simulink model "pfb_core_snbxfft"  (R2012b)
settings: Solver=FixedStepDiscrete  SolverMode=SingleTasking  StartTime=0.0  StopTime=5000  FixedStep=1  RelTol=1e-3
undefined symbols (not defined in the file or in its folder): xlipgetpartsetting
undefined symbols (not defined in the file): pfb_coeff_gen_calc
libraries: xbsIndex_r4 x3846, casper_library_misc x2, casper_library_delays x1
(part 4 of 14)

== system pfb_core_snbxfft/pfb/pfb_fir_generic/pfb_fir_coeff_gen/rom ==
  addra : Inport
  dina : Inport  Port=2
  wea : Inport  Port=3
  addrb : Inport  Port=4
  dinb : Inport  Port=5
  web : Inport  Port=6
  A_bussify : Subsystem  AncestorBlock=casper_library_flow_control/bus_create  mask(bus_create){inputNum=18}
      mask prompts: inputNum "Number of inputs:"
      mask init:
      | bus_create_init(gcb,...
      |     'inputNum', inputNum);
  B_bussify : Subsystem  AncestorBlock=casper_library_flow_control/bus_create  mask(bus_create){inputNum=18}
      mask prompts: inputNum "Number of inputs:"
      mask init:
      | bus_create_init(gcb,...
      |     'inputNum', inputNum);
  bram{0..17} (18 alike) : xbsIndex_r4/Dual Port RAM  depth=8192  initVector=getfield(get_param(gcb, 'UserData'), 'initVector')  distributed_mem=Block RAM  init_a=0  init_b=0  rst_a=off  rst_b=off  en_a=off  en_b=off  latency=8  write_mode_A=Read Before Write  write_mode_B=Read Before Write  dbl_ovrd=off  optimize=Speed  block_type=dpram
  ddina : xbsIndex_r4/Delay  rst=off  infoeditControl=Selection of Reset will increase slice count due to use of real FFs and instead of SRLs  en=off  latency=0  dbl_ovrd=off  reg_retiming=on  block_type=delay
  ddinb : xbsIndex_r4/Delay  rst=off  infoeditControl=Selection of Reset will increase slice count due to use of real FFs and instead of SRLs  en=off  latency=0  dbl_ovrd=off  reg_retiming=on  block_type=delay
  debus_addra : Subsystem  AncestorBlock=casper_library_flow_control/bus_expand  mask(bus_expand){mode=divisions of equal size, outputNum=18, outputWidth=[13 13 13 13 13 13 13 13 13 13 13 13 13 13 13 13 13 13], outputBinaryPt=[0 0 0 0 0 0 0 0 0 0 0 0 0 0 0 0 0 0], outputArithmeticType=[0 0 0 0 0 0 0 0 0 0 0 0 0 0 0 0 0 0], show_format=on, outputToWorkspace=off, variablePrefix=, outputToModelAsWell=on}
      mask prompts: outputNum "Number of outputs:"; outputWidth "Output width:"; outputBinaryPt "Output binary point position:"; outputArithmeticType "Output arithmetic type (ufix=0, fix=1, bool=2):"; show_format "Print format string?"; outputToWorkspace "Output to workspace?"; variablePrefix "Variable name prefix:"; outputToModelAsWell "Output to model as well?"
      mask help:
      | Expands a 'bus' made using a bus_create or Xilinx
      | concat block.
      | The input will be divided into the specified number
      | of outputs with the specified arithmetic types.
      | Divisions are made from most significant bit.
      mask init: same as pfb_core_snbxfft/pfb/pfb_fir_generic/bus_expand
      settings: AttributesFormatString=18 outputs: uf13.0,uf13.0,uf13.0,uf13.0,uf13.0,uf13.0,uf13.0,uf13.0,uf13.0,uf13.0,uf13.0,uf13.0,uf13.0,uf13.0,uf13.0,uf13.0,uf13.0,uf13.0,
      mask TypeOptions mode: divisions of equal size | divisions of arbitrary size
      mask Callback mode: bus_expand_callback();
      mask Callback outputWidth: bus_expand_callback();
      mask Callback outputToWorkspace: bus_expand_callback();
  debus_addrb : Subsystem  AncestorBlock=casper_library_flow_control/bus_expand  mask(bus_expand){mode=divisions of equal size, outputNum=18, outputWidth=[13 13 13 13 13 13 13 13 13 13 13 13 13 13 13 13 13 13], outputBinaryPt=[0 0 0 0 0 0 0 0 0 0 0 0 0 0 0 0 0 0], outputArithmeticType=[0 0 0 0 0 0 0 0 0 0 0 0 0 0 0 0 0 0], show_format=on, outputToWorkspace=off, variablePrefix=, outputToModelAsWell=on}
      mask prompts: outputNum "Number of outputs:"; outputWidth "Output width:"; outputBinaryPt "Output binary point position:"; outputArithmeticType "Output arithmetic type (ufix=0, fix=1, bool=2):"; show_format "Print format string?"; outputToWorkspace "Output to workspace?"; variablePrefix "Variable name prefix:"; outputToModelAsWell "Output to model as well?"
      mask help:
      | Expands a 'bus' made using a bus_create or Xilinx
      | concat block.
      | The input will be divided into the specified number
      | of outputs with the specified arithmetic types.
      | Divisions are made from most significant bit.
      mask init: same as pfb_core_snbxfft/pfb/pfb_fir_generic/bus_expand
      settings: AttributesFormatString=18 outputs: uf13.0,uf13.0,uf13.0,uf13.0,uf13.0,uf13.0,uf13.0,uf13.0,uf13.0,uf13.0,uf13.0,uf13.0,uf13.0,uf13.0,uf13.0,uf13.0,uf13.0,uf13.0,
      mask TypeOptions mode: divisions of equal size | divisions of arbitrary size
      mask Callback mode: bus_expand_callback();
      mask Callback outputWidth: bus_expand_callback();
      mask Callback outputToWorkspace: bus_expand_callback();
  debus_dina : Subsystem  AncestorBlock=casper_library_flow_control/bus_expand  mask(bus_expand){mode=divisions of arbitrary size, outputNum=1, outputWidth=[4 4 4 4 4 4 4 4 4 4 4 4 4 4 4 4 4 4], outputBinaryPt=[0 0 0 0 0 0 0 0 0 0 0 0 0 0 0 0 0 0], outputArithmeticType=[0 0 0 0 0 0 0 0 0 0 0 0 0 0 0 0 0 0], show_format=on, outputToWorkspace=off, variablePrefix=, outputToModelAsWell=on}
      mask prompts: outputNum "Number of outputs:"; outputWidth "Output width [msb ... lsb]:"; outputBinaryPt "Output binary point position [msb ... lsb]:"; outputArithmeticType "Output arithmetic type (ufix=0, fix=1, bool=2) [msb ... lsb]:"; show_format "Print format string?"; outputToWorkspace "Output to workspace?"; variablePrefix "Variable name prefix:"; outputToModelAsWell "Output to model as well?"
      mask help:
      | Expands a 'bus' made using a bus_create or Xilinx
      | concat block.
      | The input will be divided into the specified number
      | of outputs with the specified arithmetic types.
      | Divisions are made from most significant bit.
      mask init: same as pfb_core_snbxfft/pfb/pfb_fir_generic/bus_expand
      settings: AttributesFormatString=18 outputs: uf4.0,uf4.0,uf4.0,uf4.0,uf4.0,uf4.0,uf4.0,uf4.0,uf4.0,uf4.0,uf4.0,uf4.0,uf4.0,uf4.0,uf4.0,uf4.0,uf4.0,uf4.0,
      mask TypeOptions mode: divisions of equal size | divisions of arbitrary size
      mask Callback mode: bus_expand_callback();
      mask Callback outputWidth: bus_expand_callback();
      mask Callback outputToWorkspace: bus_expand_callback();
  debus_dinb : Subsystem  AncestorBlock=casper_library_flow_control/bus_expand  mask(bus_expand){mode=divisions of arbitrary size, outputNum=1, outputWidth=[4 4 4 4 4 4 4 4 4 4 4 4 4 4 4 4 4 4], outputBinaryPt=[0 0 0 0 0 0 0 0 0 0 0 0 0 0 0 0 0 0], outputArithmeticType=[0 0 0 0 0 0 0 0 0 0 0 0 0 0 0 0 0 0], show_format=on, outputToWorkspace=off, variablePrefix=, outputToModelAsWell=on}
      mask prompts: outputNum "Number of outputs:"; outputWidth "Output width [msb ... lsb]:"; outputBinaryPt "Output binary point position [msb ... lsb]:"; outputArithmeticType "Output arithmetic type (ufix=0, fix=1, bool=2) [msb ... lsb]:"; show_format "Print format string?"; outputToWorkspace "Output to workspace?"; variablePrefix "Variable name prefix:"; outputToModelAsWell "Output to model as well?"
      mask help:
      | Expands a 'bus' made using a bus_create or Xilinx
      | concat block.
      | The input will be divided into the specified number
      | of outputs with the specified arithmetic types.
      | Divisions are made from most significant bit.
      mask init: same as pfb_core_snbxfft/pfb/pfb_fir_generic/bus_expand
      settings: AttributesFormatString=18 outputs: uf4.0,uf4.0,uf4.0,uf4.0,uf4.0,uf4.0,uf4.0,uf4.0,uf4.0,uf4.0,uf4.0,uf4.0,uf4.0,uf4.0,uf4.0,uf4.0,uf4.0,uf4.0,
      mask TypeOptions mode: divisions of equal size | divisions of arbitrary size
      mask Callback mode: bus_expand_callback();
      mask Callback outputWidth: bus_expand_callback();
      mask Callback outputToWorkspace: bus_expand_callback();
  debus_wea : Subsystem  AncestorBlock=casper_library_flow_control/bus_expand  mask(bus_expand){mode=divisions of equal size, outputNum=18, outputWidth=[1 1 1 1 1 1 1 1 1 1 1 1 1 1 1 1 1 1], outputBinaryPt=[0 0 0 0 0 0 0 0 0 0 0 0 0 0 0 0 0 0], outputArithmeticType=[2 2 2 2 2 2 2 2 2 2 2 2 2 2 2 2 2 2], show_format=on, outputToWorkspace=off, variablePrefix=, outputToModelAsWell=on}
      mask prompts: outputNum "Number of outputs:"; outputWidth "Output width:"; outputBinaryPt "Output binary point position:"; outputArithmeticType "Output arithmetic type (ufix=0, fix=1, bool=2):"; show_format "Print format string?"; outputToWorkspace "Output to workspace?"; variablePrefix "Variable name prefix:"; outputToModelAsWell "Output to model as well?"
      mask help:
      | Expands a 'bus' made using a bus_create or Xilinx
      | concat block.
      | The input will be divided into the specified number
      | of outputs with the specified arithmetic types.
      | Divisions are made from most significant bit.
      mask init: same as pfb_core_snbxfft/pfb/pfb_fir_generic/bus_expand
      settings: AttributesFormatString=18 outputs: b,b,b,b,b,b,b,b,b,b,b,b,b,b,b,b,b,b,
      mask TypeOptions mode: divisions of equal size | divisions of arbitrary size
      mask Callback mode: bus_expand_callback();
      mask Callback outputWidth: bus_expand_callback();
      mask Callback outputToWorkspace: bus_expand_callback();
  debus_web : Subsystem  AncestorBlock=casper_library_flow_control/bus_expand  mask(bus_expand){mode=divisions of equal size, outputNum=18, outputWidth=[1 1 1 1 1 1 1 1 1 1 1 1 1 1 1 1 1 1], outputBinaryPt=[0 0 0 0 0 0 0 0 0 0 0 0 0 0 0 0 0 0], outputArithmeticType=[2 2 2 2 2 2 2 2 2 2 2 2 2 2 2 2 2 2], show_format=on, outputToWorkspace=off, variablePrefix=, outputToModelAsWell=on}
      mask prompts: outputNum "Number of outputs:"; outputWidth "Output width:"; outputBinaryPt "Output binary point position:"; outputArithmeticType "Output arithmetic type (ufix=0, fix=1, bool=2):"; show_format "Print format string?"; outputToWorkspace "Output to workspace?"; variablePrefix "Variable name prefix:"; outputToModelAsWell "Output to model as well?"
      mask help:
      | Expands a 'bus' made using a bus_create or Xilinx
      | concat block.
      | The input will be divided into the specified number
      | of outputs with the specified arithmetic types.
      | Divisions are made from most significant bit.
      mask init: same as pfb_core_snbxfft/pfb/pfb_fir_generic/bus_expand
      settings: AttributesFormatString=18 outputs: b,b,b,b,b,b,b,b,b,b,b,b,b,b,b,b,b,b,
      mask TypeOptions mode: divisions of equal size | divisions of arbitrary size
      mask Callback mode: bus_expand_callback();
      mask Callback outputWidth: bus_expand_callback();
      mask Callback outputToWorkspace: bus_expand_callback();
  rep_addra : Subsystem  AncestorBlock=casper_library_bus/bus_replicate  mask(bus_replicate){replication=18, latency=9, misc=off, implementation=core}
      mask prompts: replication "replication factor"; misc "misc support"; implementation "delay implementation"
      mask help: Output bus formed by replicating input bus a number of times
      mask init:
      | bus_replicate_init(gcb, ...
      |     'replication', replication, ...
      |     'latency', latency, ...
      |     'implementation', implementation, ...
      |     'misc', misc);
      mask TypeOptions implementation: core | behavioral
  rep_addrb : Subsystem  AncestorBlock=casper_library_bus/bus_replicate  mask(bus_replicate){replication=18, latency=9, misc=off, implementation=core}
      mask prompts: replication "replication factor"; misc "misc support"; implementation "delay implementation"
      mask help: Output bus formed by replicating input bus a number of times
      mask init:
      | bus_replicate_init(gcb, ...
      |     'replication', replication, ...
      |     'latency', latency, ...
      |     'implementation', implementation, ...
      |     'misc', misc);
      mask TypeOptions implementation: core | behavioral
  rep_wea : Subsystem  AncestorBlock=casper_library_bus/bus_replicate  mask(bus_replicate){replication=18, latency=0, misc=off, implementation=behavioral}
      mask prompts: replication "replication factor"; misc "misc support"; implementation "delay implementation"
      mask help: Output bus formed by replicating input bus a number of times
      mask init:
      | bus_replicate_init(gcb, ...
      |     'replication', replication, ...
      |     'latency', latency, ...
      |     'implementation', implementation, ...
      |     'misc', misc);
      mask TypeOptions implementation: core | behavioral
  rep_web : Subsystem  AncestorBlock=casper_library_bus/bus_replicate  mask(bus_replicate){replication=18, latency=0, misc=off, implementation=behavioral}
      mask prompts: replication "replication factor"; misc "misc support"; implementation "delay implementation"
      mask help: Output bus formed by replicating input bus a number of times
      mask init:
      | bus_replicate_init(gcb, ...
      |     'replication', replication, ...
      |     'latency', latency, ...
      |     'implementation', implementation, ...
      |     'misc', misc);
      mask TypeOptions implementation: core | behavioral
  A : Outport
  B : Outport  Port=2
  wires:
  addra/1 -> rep_addra/1(in)
  dina/1 -> ddina/1
  wea/1 -> rep_wea/1(in)
  addrb/1 -> rep_addrb/1(in)
  dinb/1 -> ddinb/1
  web/1 -> rep_web/1(in)
  rep_addra/1(out) -> debus_addra/1(bus_in)
  ddina/1 -> debus_dina/1(bus_in)
  rep_wea/1(out) -> debus_wea/1(bus_in)
  rep_addrb/1(out) -> debus_addrb/1(bus_in)
  ddinb/1 -> debus_dinb/1(bus_in)
  rep_web/1(out) -> debus_web/1(bus_in)
  debus_addra/1(msb_out18) -> bram0/1
  debus_dina/1(msb_out18) -> bram0/2
  debus_wea/1(msb_out18) -> bram0/3
  debus_addrb/1(msb_out18) -> bram0/4
  debus_dinb/1(msb_out18) -> bram0/5
  debus_web/1(msb_out18) -> bram0/6
  debus_addra/2(out17) -> bram1/1
  debus_dina/2(out17) -> bram1/2
  debus_wea/2(out17) -> bram1/3
  debus_addrb/2(out17) -> bram1/4
  debus_dinb/2(out17) -> bram1/5
  debus_web/2(out17) -> bram1/6
  debus_addra/3(out16) -> bram2/1
  debus_dina/3(out16) -> bram2/2
  debus_wea/3(out16) -> bram2/3
  debus_addrb/3(out16) -> bram2/4
  debus_dinb/3(out16) -> bram2/5
  debus_web/3(out16) -> bram2/6
  debus_addra/4(out15) -> bram3/1
  debus_dina/4(out15) -> bram3/2
  debus_wea/4(out15) -> bram3/3
  debus_addrb/4(out15) -> bram3/4
  debus_dinb/4(out15) -> bram3/5
  debus_web/4(out15) -> bram3/6
  debus_addra/5(out14) -> bram4/1
  debus_dina/5(out14) -> bram4/2
  debus_wea/5(out14) -> bram4/3
  debus_addrb/5(out14) -> bram4/4
  debus_dinb/5(out14) -> bram4/5
  debus_web/5(out14) -> bram4/6
  debus_addra/6(out13) -> bram5/1
  debus_dina/6(out13) -> bram5/2
  debus_wea/6(out13) -> bram5/3
  debus_addrb/6(out13) -> bram5/4
  debus_dinb/6(out13) -> bram5/5
  debus_web/6(out13) -> bram5/6
  debus_addra/7(out12) -> bram6/1
  debus_dina/7(out12) -> bram6/2
  debus_wea/7(out12) -> bram6/3
  debus_addrb/7(out12) -> bram6/4
  debus_dinb/7(out12) -> bram6/5
  debus_web/7(out12) -> bram6/6
  debus_addra/8(out11) -> bram7/1
  debus_dina/8(out11) -> bram7/2
  debus_wea/8(out11) -> bram7/3
  debus_addrb/8(out11) -> bram7/4
  debus_dinb/8(out11) -> bram7/5
  debus_web/8(out11) -> bram7/6
  debus_addra/9(out10) -> bram8/1
  debus_dina/9(out10) -> bram8/2
  debus_wea/9(out10) -> bram8/3
  debus_addrb/9(out10) -> bram8/4
  debus_dinb/9(out10) -> bram8/5
  debus_web/9(out10) -> bram8/6
  debus_addra/10(out9) -> bram9/1
  debus_dina/10(out9) -> bram9/2
  debus_wea/10(out9) -> bram9/3
  debus_addrb/10(out9) -> bram9/4
  debus_dinb/10(out9) -> bram9/5
  debus_web/10(out9) -> bram9/6
  debus_addra/11(out8) -> bram10/1
  debus_dina/11(out8) -> bram10/2
  debus_wea/11(out8) -> bram10/3
  debus_addrb/11(out8) -> bram10/4
  debus_dinb/11(out8) -> bram10/5
  debus_web/11(out8) -> bram10/6
  debus_addra/12(out7) -> bram11/1
  debus_dina/12(out7) -> bram11/2
  debus_wea/12(out7) -> bram11/3
  debus_addrb/12(out7) -> bram11/4
  debus_dinb/12(out7) -> bram11/5
  debus_web/12(out7) -> bram11/6
  debus_addra/13(out6) -> bram12/1
  debus_dina/13(out6) -> bram12/2
  debus_wea/13(out6) -> bram12/3
  debus_addrb/13(out6) -> bram12/4
  debus_dinb/13(out6) -> bram12/5
  debus_web/13(out6) -> bram12/6
  debus_addra/14(out5) -> bram13/1
  debus_dina/14(out5) -> bram13/2
  debus_wea/14(out5) -> bram13/3
  debus_addrb/14(out5) -> bram13/4
  debus_dinb/14(out5) -> bram13/5
  debus_web/14(out5) -> bram13/6
  debus_addra/15(out4) -> bram14/1
  debus_dina/15(out4) -> bram14/2
  debus_wea/15(out4) -> bram14/3
  debus_addrb/15(out4) -> bram14/4
  debus_dinb/15(out4) -> bram14/5
  debus_web/15(out4) -> bram14/6
  debus_addra/16(out3) -> bram15/1
  debus_dina/16(out3) -> bram15/2
  debus_wea/16(out3) -> bram15/3
  debus_addrb/16(out3) -> bram15/4
  debus_dinb/16(out3) -> bram15/5
  debus_web/16(out3) -> bram15/6
  debus_addra/17(out2) -> bram16/1
  debus_dina/17(out2) -> bram16/2
  debus_wea/17(out2) -> bram16/3
  debus_addrb/17(out2) -> bram16/4
  debus_dinb/17(out2) -> bram16/5
  debus_web/17(out2) -> bram16/6
  debus_addra/18(lsb_out1) -> bram17/1
  debus_dina/18(lsb_out1) -> bram17/2
  debus_wea/18(lsb_out1) -> bram17/3
  debus_addrb/18(lsb_out1) -> bram17/4
  debus_dinb/18(lsb_out1) -> bram17/5
  debus_web/18(lsb_out1) -> bram17/6
  bram0/1 -> A_bussify/1(in1)
  bram0/2 -> B_bussify/1(in1)
  bram1/1 -> A_bussify/2(in2)
  bram1/2 -> B_bussify/2(in2)
  bram2/1 -> A_bussify/3(in3)
  bram2/2 -> B_bussify/3(in3)
  bram3/1 -> A_bussify/4(in4)
  bram3/2 -> B_bussify/4(in4)
  bram4/1 -> A_bussify/5(in5)
  bram4/2 -> B_bussify/5(in5)
  bram5/1 -> A_bussify/6(in6)
  bram5/2 -> B_bussify/6(in6)
  bram6/1 -> A_bussify/7(in7)
  bram6/2 -> B_bussify/7(in7)
  bram7/1 -> A_bussify/8(in8)
  bram7/2 -> B_bussify/8(in8)
  bram8/1 -> A_bussify/9(in9)
  bram8/2 -> B_bussify/9(in9)
  bram9/1 -> A_bussify/10(in10)
  bram9/2 -> B_bussify/10(in10)
  bram10/1 -> A_bussify/11(in11)
  bram10/2 -> B_bussify/11(in11)
  bram11/1 -> A_bussify/12(in12)
  bram11/2 -> B_bussify/12(in12)
  bram12/1 -> A_bussify/13(in13)
  bram12/2 -> B_bussify/13(in13)
  bram13/1 -> A_bussify/14(in14)
  bram13/2 -> B_bussify/14(in14)
  bram14/1 -> A_bussify/15(in15)
  bram14/2 -> B_bussify/15(in15)
  bram15/1 -> A_bussify/16(in16)
  bram15/2 -> B_bussify/16(in16)
  bram16/1 -> A_bussify/17(in17)
  bram16/2 -> B_bussify/17(in17)
  bram17/1 -> A_bussify/18(in18)
  bram17/2 -> B_bussify/18(in18)
  A_bussify/1(bus_out) -> A/1
  B_bussify/1(bus_out) -> B/1

== system pfb_core_snbxfft/pfb/pfb_fir_generic/pfb_fir_taps/bus_madd ==
  a : Inport
  b : Inport  Port=2
  c : Inport  Port=3
  en : Inport  Port=4
  a*b+c_bussify : Subsystem  AncestorBlock=casper_library_flow_control/bus_create  mask(bus_create){inputNum=32}
      mask prompts: inputNum "Number of inputs:"
      mask init:
      | bus_create_init(gcb,...
      |     'inputNum', inputNum);
  a_debus : Subsystem  AncestorBlock=casper_library_flow_control/bus_expand  mask(bus_expand){mode=divisions of arbitrary size, outputNum=1, outputWidth=[18 18 18 18 18 18 18 18 18 18 18 18 18 18 18 18 18 18 18 18 18 18 18 18 18 18 18 18 18 18 18 18], outputBinaryPt=[17 17 17 17 17 17 17 17 17 17 17 17 17 17 17 17 17 17 17 17 17 17 17 17 17 17 17 17 17 17 17 17], outputArithmeticType=[1 1 1 1 1 1 1 1 1 1 1 1 1 1 1 1 1 1 1 1 1 1 1 1 1 1 1 1 1 1 1 1], show_format=on, outputToWorkspace=off, variablePrefix=, outputToModelAsWell=on}
      mask prompts: outputNum "Number of outputs:"; outputWidth "Output width [msb ... lsb]:"; outputBinaryPt "Output binary point position [msb ... lsb]:"; outputArithmeticType "Output arithmetic type (ufix=0, fix=1, bool=2) [msb ... lsb]:"; show_format "Print format string?"; outputToWorkspace "Output to workspace?"; variablePrefix "Variable name prefix:"; outputToModelAsWell "Output to model as well?"
      mask help:
      | Expands a 'bus' made using a bus_create or Xilinx
      | concat block.
      | The input will be divided into the specified number
      | of outputs with the specified arithmetic types.
      | Divisions are made from most significant bit.
      mask init: same as pfb_core_snbxfft/pfb/pfb_fir_generic/bus_expand
      settings: AttributesFormatString=32 outputs: f18.17,f18.17,f18.17,f18.17,f18.17,f18.17,f18.17,f18.17,f18.17,f18.17,f18.17,f18.17,f18.17,f18.17,f18.17,f18.17,f18.17,f18.17,f18.17,f18.17,f18.17,f18.17,f18.17,f18.17,f18.17,f18.17,f18.17,f18.17,f18.17,f18.17,f18.17,f18.17,
      mask TypeOptions mode: divisions of equal size | divisions of arbitrary size
      mask Callback mode: bus_expand_callback();
      mask Callback outputWidth: bus_expand_callback();
      mask Callback outputToWorkspace: bus_expand_callback();
  addsub{1..4} (4 alike) : xbsIndex_r4/AddSub  mode=Addition  use_carryin=off  use_carryout=off  en=on  latency=2  precision=User Defined  arith_type="Signed  (2's comp)"  n_bits=36  bin_pt=34  quantization=Truncate  overflow=Wrap  dbl_ovrd=off  use_behavioral_HDL=on  hw_selection=Fabric  pipelined=on  block_type=addsub
  addsub{9..12} (4 alike) : xbsIndex_r4/AddSub  mode=Addition  use_carryin=off  use_carryout=off  en=on  latency=2  precision=User Defined  arith_type="Signed  (2's comp)"  n_bits=38  bin_pt=34  quantization=Truncate  overflow=Wrap  dbl_ovrd=off  use_behavioral_HDL=on  hw_selection=Fabric  pipelined=on  block_type=addsub
  addsub{13..16} (4 alike) : xbsIndex_r4/AddSub  mode=Addition  use_carryin=off  use_carryout=off  en=on  latency=2  precision=User Defined  arith_type="Signed  (2's comp)"  n_bits=39  bin_pt=34  quantization=Truncate  overflow=Wrap  dbl_ovrd=off  use_behavioral_HDL=on  hw_selection=Fabric  pipelined=on  block_type=addsub
  addsub{17..20} (4 alike) : xbsIndex_r4/AddSub  mode=Addition  use_carryin=off  use_carryout=off  en=on  latency=2  precision=User Defined  arith_type="Signed  (2's comp)"  n_bits=40  bin_pt=34  quantization=Truncate  overflow=Wrap  dbl_ovrd=off  use_behavioral_HDL=on  hw_selection=Fabric  pipelined=on  block_type=addsub
  addsub{21..24} (4 alike) : xbsIndex_r4/AddSub  mode=Addition  use_carryin=off  use_carryout=off  en=on  latency=2  precision=User Defined  arith_type="Signed  (2's comp)"  n_bits=41  bin_pt=34  quantization=Truncate  overflow=Wrap  dbl_ovrd=off  use_behavioral_HDL=on  hw_selection=Fabric  pipelined=on  block_type=addsub
  addsub{25..28} (4 alike) : xbsIndex_r4/AddSub  mode=Addition  use_carryin=off  use_carryout=off  en=on  latency=2  precision=User Defined  arith_type="Signed  (2's comp)"  n_bits=42  bin_pt=34  quantization=Truncate  overflow=Wrap  dbl_ovrd=off  use_behavioral_HDL=on  hw_selection=Fabric  pipelined=on  block_type=addsub
  addsub{29..32} (4 alike) : xbsIndex_r4/AddSub  mode=Addition  use_carryin=off  use_carryout=off  en=on  latency=2  precision=User Defined  arith_type="Signed  (2's comp)"  n_bits=43  bin_pt=34  quantization=Truncate  overflow=Wrap  dbl_ovrd=off  use_behavioral_HDL=on  hw_selection=Fabric  pipelined=on  block_type=addsub
  addsub{5..8} (4 alike) : xbsIndex_r4/AddSub  mode=Addition  use_carryin=off  use_carryout=off  en=on  latency=2  precision=User Defined  arith_type="Signed  (2's comp)"  n_bits=37  bin_pt=34  quantization=Truncate  overflow=Wrap  dbl_ovrd=off  use_behavioral_HDL=on  hw_selection=Fabric  pipelined=on  block_type=addsub
  b_debus : Subsystem  AncestorBlock=casper_library_flow_control/bus_expand  mask(bus_expand){mode=divisions of arbitrary size, outputNum=1, outputWidth=[18 18 18 18 18 18 18 18 18 18 18 18 18 18 18 18 18 18 18 18 18 18 18 18 18 18 18 18 18 18 18 18], outputBinaryPt=[17 17 17 17 17 17 17 17 17 17 17 17 17 17 17 17 17 17 17 17 17 17 17 17 17 17 17 17 17 17 17 17], outputArithmeticType=[1 1 1 1 1 1 1 1 1 1 1 1 1 1 1 1 1 1 1 1 1 1 1 1 1 1 1 1 1 1 1 1], show_format=on, outputToWorkspace=off, variablePrefix=, outputToModelAsWell=on}
      mask prompts: outputNum "Number of outputs:"; outputWidth "Output width [msb ... lsb]:"; outputBinaryPt "Output binary point position [msb ... lsb]:"; outputArithmeticType "Output arithmetic type (ufix=0, fix=1, bool=2) [msb ... lsb]:"; show_format "Print format string?"; outputToWorkspace "Output to workspace?"; variablePrefix "Variable name prefix:"; outputToModelAsWell "Output to model as well?"
      mask help:
      | Expands a 'bus' made using a bus_create or Xilinx
      | concat block.
      | The input will be divided into the specified number
      | of outputs with the specified arithmetic types.
      | Divisions are made from most significant bit.
      mask init: same as pfb_core_snbxfft/pfb/pfb_fir_generic/bus_expand
      settings: AttributesFormatString=32 outputs: f18.17,f18.17,f18.17,f18.17,f18.17,f18.17,f18.17,f18.17,f18.17,f18.17,f18.17,f18.17,f18.17,f18.17,f18.17,f18.17,f18.17,f18.17,f18.17,f18.17,f18.17,f18.17,f18.17,f18.17,f18.17,f18.17,f18.17,f18.17,f18.17,f18.17,f18.17,f18.17,
      mask TypeOptions mode: divisions of equal size | divisions of arbitrary size
      mask Callback mode: bus_expand_callback();
      mask Callback outputWidth: bus_expand_callback();
      mask Callback outputToWorkspace: bus_expand_callback();
  c_debus : Subsystem  AncestorBlock=casper_library_flow_control/bus_expand  mask(bus_expand){mode=divisions of arbitrary size, outputNum=1, outputWidth=[36 36 36 36 36 36 36 36 37 37 37 37 38 38 38 38 39 39 39 39 40 40 40 40 41 41 41 41 42 42 42 42], outputBinaryPt=[34 34 34 34 34 34 34 34 34 34 34 34 34 34 34 34 34 34 34 34 34 34 34 34 34 34 34 34 34 34 34 34], outputArithmeticType=[1 1 1 1 1 1 1 1 1 1 1 1 1 1 1 1 1 1 1 1 1 1 1 1 1 1 1 1 1 1 1 1], show_format=on, outputToWorkspace=off, variablePrefix=, outputToModelAsWell=on}
      mask prompts: outputNum "Number of outputs:"; outputWidth "Output width [msb ... lsb]:"; outputBinaryPt "Output binary point position [msb ... lsb]:"; outputArithmeticType "Output arithmetic type (ufix=0, fix=1, bool=2) [msb ... lsb]:"; show_format "Print format string?"; outputToWorkspace "Output to workspace?"; variablePrefix "Variable name prefix:"; outputToModelAsWell "Output to model as well?"
      mask help:
      | Expands a 'bus' made using a bus_create or Xilinx
      | concat block.
      | The input will be divided into the specified number
      | of outputs with the specified arithmetic types.
      | Divisions are made from most significant bit.
      mask init: same as pfb_core_snbxfft/pfb/pfb_fir_generic/bus_expand
      settings: AttributesFormatString=32 outputs: f36.34,f36.34,f36.34,f36.34,f36.34,f36.34,f36.34,f36.34,f37.34,f37.34,f37.34,f37.34,f38.34,f38.34,f38.34,f38.34,f39.34,f39.34,f39.34,f39.34,f40.34,f40.34,f40.34,f40.34,f41.34,f41.34,f41.34,f41.34,f42.34,f42.34,f42.34,f42.34,
      mask TypeOptions mode: divisions of equal size | divisions of arbitrary size
      mask Callback mode: bus_expand_callback();
      mask Callback outputWidth: bus_expand_callback();
      mask Callback outputToWorkspace: bus_expand_callback();
  den0 : xbsIndex_r4/Delay  rst=off  infoeditControl=Selection of Reset will increase slice count due to use of real FFs and instead of SRLs  en=off  latency=3  dbl_ovrd=off  reg_retiming=on  block_type=delay
  den1 : xbsIndex_r4/Delay  rst=off  infoeditControl=Selection of Reset will increase slice count due to use of real FFs and instead of SRLs  en=off  latency=1  dbl_ovrd=off  reg_retiming=on  block_type=delay
  den2 : xbsIndex_r4/Delay  rst=off  infoeditControl=Selection of Reset will increase slice count due to use of real FFs and instead of SRLs  en=off  latency=2  dbl_ovrd=off  reg_retiming=on  block_type=delay
  en_debus1 : Subsystem  AncestorBlock=casper_library_flow_control/bus_expand  mask(bus_expand){mode=divisions of equal size, outputNum=32, outputWidth=1, outputBinaryPt=0, outputArithmeticType=2, show_format=on, outputToWorkspace=off, variablePrefix=, outputToModelAsWell=on}
      mask prompts: outputNum "Number of outputs:"; outputWidth "Output width:"; outputBinaryPt "Output binary point position:"; outputArithmeticType "Output arithmetic type (ufix=0, fix=1, bool=2):"; show_format "Print format string?"; outputToWorkspace "Output to workspace?"; variablePrefix "Variable name prefix:"; outputToModelAsWell "Output to model as well?"
      mask help:
      | Expands a 'bus' made using a bus_create or Xilinx
      | concat block.
      | The input will be divided into the specified number
      | of outputs with the specified arithmetic types.
      | Divisions are made from most significant bit.
      mask init: same as pfb_core_snbxfft/pfb/pfb_fir_generic/bus_expand
      settings: AttributesFormatString=32 outputs: b,b,b,b,b,b,b,b,b,b,b,b,b,b,b,b,b,b,b,b,b,b,b,b,b,b,b,b,b,b,b,b,
      mask TypeOptions mode: divisions of equal size | divisions of arbitrary size
      mask Callback mode: bus_expand_callback();
      mask Callback outputWidth: bus_expand_callback();
      mask Callback outputToWorkspace: bus_expand_callback();
  mult{1..32} (32 alike) : xbsIndex_r4/Mult  precision=Full  arith_type="Signed  (2's comp)"  n_bits=16  bin_pt=14  quantization=Truncate  overflow=Wrap  en=off  latency=3  dbl_ovrd=off  use_behavioral_HDL=on  opt=Speed  use_embedded=off  optimum_pipeline=off  pipeline=on  use_rpm=on  placement_style=Triangular  block_type=mult
  repa : Subsystem  AncestorBlock=casper_library_bus/bus_replicate  mask(bus_replicate){replication=1, latency=1, misc=off, implementation=core}
      mask prompts: replication "replication factor"; misc "misc support"; implementation "delay implementation"
      mask help: Output bus formed by replicating input bus a number of times
      mask init:
      | bus_replicate_init(gcb, ...
      |     'replication', replication, ...
      |     'latency', latency, ...
      |     'implementation', implementation, ...
      |     'misc', misc);
      mask TypeOptions implementation: core | behavioral
  repb : Subsystem  AncestorBlock=casper_library_bus/bus_replicate  mask(bus_replicate){replication=1, latency=1, misc=off, implementation=core}
      mask prompts: replication "replication factor"; misc "misc support"; implementation "delay implementation"
      mask help: Output bus formed by replicating input bus a number of times
      mask init:
      | bus_replicate_init(gcb, ...
      |     'replication', replication, ...
      |     'latency', latency, ...
      |     'implementation', implementation, ...
      |     'misc', misc);
      mask TypeOptions implementation: core | behavioral
  repen1 : Subsystem  AncestorBlock=casper_library_bus/bus_replicate  mask(bus_replicate){replication=32, latency=4, misc=off, implementation=core}
      mask prompts: replication "replication factor"; misc "misc support"; implementation "delay implementation"
      mask help: Output bus formed by replicating input bus a number of times
      mask init:
      | bus_replicate_init(gcb, ...
      |     'replication', replication, ...
      |     'latency', latency, ...
      |     'implementation', implementation, ...
      |     'misc', misc);
      mask TypeOptions implementation: core | behavioral
  a*b+c : Outport
  dvalid : Outport  Port=2
  wires:
  den2/1 -> dvalid/1
  a*b+c_bussify/1(bus_out) -> a*b+c/1
  addsub32/1 -> a*b+c_bussify/32(in32)
  addsub31/1 -> a*b+c_bussify/31(in31)
  addsub30/1 -> a*b+c_bussify/30(in30)
  addsub29/1 -> a*b+c_bussify/29(in29)
  addsub28/1 -> a*b+c_bussify/28(in28)
  addsub27/1 -> a*b+c_bussify/27(in27)
  addsub26/1 -> a*b+c_bussify/26(in26)
  addsub25/1 -> a*b+c_bussify/25(in25)
  addsub24/1 -> a*b+c_bussify/24(in24)
  addsub23/1 -> a*b+c_bussify/23(in23)
  addsub22/1 -> a*b+c_bussify/22(in22)
  addsub21/1 -> a*b+c_bussify/21(in21)
  addsub20/1 -> a*b+c_bussify/20(in20)
  addsub19/1 -> a*b+c_bussify/19(in19)
  addsub18/1 -> a*b+c_bussify/18(in18)
  addsub17/1 -> a*b+c_bussify/17(in17)
  addsub16/1 -> a*b+c_bussify/16(in16)
  addsub15/1 -> a*b+c_bussify/15(in15)
  addsub14/1 -> a*b+c_bussify/14(in14)
  addsub13/1 -> a*b+c_bussify/13(in13)
  addsub12/1 -> a*b+c_bussify/12(in12)
  addsub11/1 -> a*b+c_bussify/11(in11)
  addsub10/1 -> a*b+c_bussify/10(in10)
  addsub9/1 -> a*b+c_bussify/9(in9)
  addsub8/1 -> a*b+c_bussify/8(in8)
  addsub7/1 -> a*b+c_bussify/7(in7)
  addsub6/1 -> a*b+c_bussify/6(in6)
  addsub5/1 -> a*b+c_bussify/5(in5)
  addsub4/1 -> a*b+c_bussify/4(in4)
  addsub3/1 -> a*b+c_bussify/3(in3)
  addsub2/1 -> a*b+c_bussify/2(in2)
  addsub1/1 -> a*b+c_bussify/1(in1)
  den1/1 -> den2/1
  en_debus1/32(lsb_out1) -> addsub32/3
  c_debus/32(lsb_out1) -> addsub32/2
  mult32/1 -> addsub32/1
  en_debus1/31(out2) -> addsub31/3
  c_debus/31(out2) -> addsub31/2
  mult31/1 -> addsub31/1
  en_debus1/30(out3) -> addsub30/3
  c_debus/30(out3) -> addsub30/2
  mult30/1 -> addsub30/1
  en_debus1/29(out4) -> addsub29/3
  c_debus/29(out4) -> addsub29/2
  mult29/1 -> addsub29/1
  en_debus1/28(out5) -> addsub28/3
  c_debus/28(out5) -> addsub28/2
  mult28/1 -> addsub28/1
  en_debus1/27(out6) -> addsub27/3
  c_debus/27(out6) -> addsub27/2
  mult27/1 -> addsub27/1
  en_debus1/26(out7) -> addsub26/3
  c_debus/26(out7) -> addsub26/2
  mult26/1 -> addsub26/1
  en_debus1/25(out8) -> addsub25/3
  c_debus/25(out8) -> addsub25/2
  mult25/1 -> addsub25/1
  en_debus1/24(out9) -> addsub24/3
  c_debus/24(out9) -> addsub24/2
  mult24/1 -> addsub24/1
  en_debus1/23(out10) -> addsub23/3
  c_debus/23(out10) -> addsub23/2
  mult23/1 -> addsub23/1
  en_debus1/22(out11) -> addsub22/3
  c_debus/22(out11) -> addsub22/2
  mult22/1 -> addsub22/1
  en_debus1/21(out12) -> addsub21/3
  c_debus/21(out12) -> addsub21/2
  mult21/1 -> addsub21/1
  en_debus1/20(out13) -> addsub20/3
  c_debus/20(out13) -> addsub20/2
  mult20/1 -> addsub20/1
  en_debus1/19(out14) -> addsub19/3
  c_debus/19(out14) -> addsub19/2
  mult19/1 -> addsub19/1
  en_debus1/18(out15) -> addsub18/3
  c_debus/18(out15) -> addsub18/2
  mult18/1 -> addsub18/1
  en_debus1/17(out16) -> addsub17/3
  c_debus/17(out16) -> addsub17/2
  mult17/1 -> addsub17/1
  en_debus1/16(out17) -> addsub16/3
  c_debus/16(out17) -> addsub16/2
  mult16/1 -> addsub16/1
  en_debus1/15(out18) -> addsub15/3
  c_debus/15(out18) -> addsub15/2
  mult15/1 -> addsub15/1
  en_debus1/14(out19) -> addsub14/3
  c_debus/14(out19) -> addsub14/2
  mult14/1 -> addsub14/1
  en_debus1/13(out20) -> addsub13/3
  c_debus/13(out20) -> addsub13/2
  mult13/1 -> addsub13/1
  en_debus1/12(out21) -> addsub12/3
  c_debus/12(out21) -> addsub12/2
  mult12/1 -> addsub12/1
  en_debus1/11(out22) -> addsub11/3
  c_debus/11(out22) -> addsub11/2
  mult11/1 -> addsub11/1
  en_debus1/10(out23) -> addsub10/3
  c_debus/10(out23) -> addsub10/2
  mult10/1 -> addsub10/1
  en_debus1/9(out24) -> addsub9/3
  c_debus/9(out24) -> addsub9/2
  mult9/1 -> addsub9/1
  en_debus1/8(out25) -> addsub8/3
  c_debus/8(out25) -> addsub8/2
  mult8/1 -> addsub8/1
  en_debus1/7(out26) -> addsub7/3
  c_debus/7(out26) -> addsub7/2
  mult7/1 -> addsub7/1
  en_debus1/6(out27) -> addsub6/3
  c_debus/6(out27) -> addsub6/2
  mult6/1 -> addsub6/1
  en_debus1/5(out28) -> addsub5/3
  c_debus/5(out28) -> addsub5/2
  mult5/1 -> addsub5/1
  en_debus1/4(out29) -> addsub4/3
  c_debus/4(out29) -> addsub4/2
  mult4/1 -> addsub4/1
  en_debus1/3(out30) -> addsub3/3
  c_debus/3(out30) -> addsub3/2
  mult3/1 -> addsub3/1
  en_debus1/2(out31) -> addsub2/3
  c_debus/2(out31) -> addsub2/2
  mult2/1 -> addsub2/1
  en_debus1/1(msb_out32) -> addsub1/3
  c_debus/1(msb_out32) -> addsub1/2
  mult1/1 -> addsub1/1
  repen1/1(out) -> en_debus1/1(bus_in)
  c/1 -> c_debus/1(bus_in)
  den0/1 -> den1/1
  en/1 -> repen1/1(in), den0/1
  b_debus/32(lsb_out1) -> mult32/2
  a_debus/32(lsb_out1) -> mult32/1
  b_debus/31(out2) -> mult31/2
  a_debus/31(out2) -> mult31/1
  b_debus/30(out3) -> mult30/2
  a_debus/30(out3) -> mult30/1
  b_debus/29(out4) -> mult29/2
  a_debus/29(out4) -> mult29/1
  b_debus/28(out5) -> mult28/2
  a_debus/28(out5) -> mult28/1
  b_debus/27(out6) -> mult27/2
  a_debus/27(out6) -> mult27/1
  b_debus/26(out7) -> mult26/2
  a_debus/26(out7) -> mult26/1
  b_debus/25(out8) -> mult25/2
  a_debus/25(out8) -> mult25/1
  b_debus/24(out9) -> mult24/2
  a_debus/24(out9) -> mult24/1
  b_debus/23(out10) -> mult23/2
  a_debus/23(out10) -> mult23/1
  b_debus/22(out11) -> mult22/2
  a_debus/22(out11) -> mult22/1
  b_debus/21(out12) -> mult21/2
  a_debus/21(out12) -> mult21/1
  b_debus/20(out13) -> mult20/2
  a_debus/20(out13) -> mult20/1
  b_debus/19(out14) -> mult19/2
  a_debus/19(out14) -> mult19/1
  b_debus/18(out15) -> mult18/2
  a_debus/18(out15) -> mult18/1
  b_debus/17(out16) -> mult17/2
  a_debus/17(out16) -> mult17/1
  b_debus/16(out17) -> mult16/2
  a_debus/16(out17) -> mult16/1
  b_debus/15(out18) -> mult15/2
  a_debus/15(out18) -> mult15/1
  b_debus/14(out19) -> mult14/2
  a_debus/14(out19) -> mult14/1
  b_debus/13(out20) -> mult13/2
  a_debus/13(out20) -> mult13/1
  b_debus/12(out21) -> mult12/2
  a_debus/12(out21) -> mult12/1
  b_debus/11(out22) -> mult11/2
  a_debus/11(out22) -> mult11/1
  b_debus/10(out23) -> mult10/2
  a_debus/10(out23) -> mult10/1
  b_debus/9(out24) -> mult9/2
  a_debus/9(out24) -> mult9/1
  b_debus/8(out25) -> mult8/2
  a_debus/8(out25) -> mult8/1
  b_debus/7(out26) -> mult7/2
  a_debus/7(out26) -> mult7/1
  b_debus/6(out27) -> mult6/2
  a_debus/6(out27) -> mult6/1
  b_debus/5(out28) -> mult5/2
  a_debus/5(out28) -> mult5/1
  b_debus/4(out29) -> mult4/2
  a_debus/4(out29) -> mult4/1
  b_debus/3(out30) -> mult3/2
  a_debus/3(out30) -> mult3/1
  b_debus/2(out31) -> mult2/2
  a_debus/2(out31) -> mult2/1
  b_debus/1(msb_out32) -> mult1/2
  a_debus/1(msb_out32) -> mult1/1
  repb/1(out) -> b_debus/1(bus_in)
  repa/1(out) -> a_debus/1(bus_in)
  b/1 -> repb/1(in)
  a/1 -> repa/1(in)

== system pfb_core_snbxfft/pfb/pfb_fir_generic/pfb_fir_taps/ddata0 ==
  din : Inport
  en : Inport  Port=2
  del{1..12} (12 alike) : xbsIndex_r4/Delay  rst=off  infoeditControl=Selection of Reset will increase slice count due to use of real FFs and instead of SRLs  en=on  latency=2  dbl_ovrd=off  reg_retiming=on  block_type=delay
  din_expand : Subsystem  AncestorBlock=casper_library_flow_control/bus_expand  mask(bus_expand){mode=divisions of arbitrary size, outputNum=1, outputWidth=[36  36  36  36  36  36  36  36  36  36  36  36], outputBinaryPt=[0  0  0  0  0  0  0  0  0  0  0  0], outputArithmeticType=[0  0  0  0  0  0  0  0  0  0  0  0], show_format=on, outputToWorkspace=off, variablePrefix=, outputToModelAsWell=on}
      mask prompts: outputNum "Number of outputs:"; outputWidth "Output width [msb ... lsb]:"; outputBinaryPt "Output binary point position [msb ... lsb]:"; outputArithmeticType "Output arithmetic type (ufix=0, fix=1, bool=2) [msb ... lsb]:"; show_format "Print format string?"; outputToWorkspace "Output to workspace?"; variablePrefix "Variable name prefix:"; outputToModelAsWell "Output to model as well?"
      mask help:
      | Expands a 'bus' made using a bus_create or Xilinx
      | concat block.
      | The input will be divided into the specified number
      | of outputs with the specified arithmetic types.
      | Divisions are made from most significant bit.
      mask init: same as pfb_core_snbxfft/pfb/pfb_fir_generic/bus_expand
      settings: AttributesFormatString=12 outputs: uf36.0,uf36.0,uf36.0,uf36.0,uf36.0,uf36.0,uf36.0,uf36.0,uf36.0,uf36.0,uf36.0,uf36.0,
      mask TypeOptions mode: divisions of equal size | divisions of arbitrary size
      mask Callback mode: bus_expand_callback();
      mask Callback outputWidth: bus_expand_callback();
      mask Callback outputToWorkspace: bus_expand_callback();
  dout_compress : Subsystem  AncestorBlock=casper_library_flow_control/bus_create  mask(bus_create){inputNum=12}
      mask prompts: inputNum "Number of inputs:"
      mask init:
      | bus_create_init(gcb,...
      |     'inputNum', inputNum);
  en_expand : Subsystem  AncestorBlock=casper_library_flow_control/bus_expand  mask(bus_expand){mode=divisions of equal size, outputNum=12, outputWidth=1, outputBinaryPt=0, outputArithmeticType=2, show_format=on, outputToWorkspace=off, variablePrefix=, outputToModelAsWell=on}
      mask prompts: outputNum "Number of outputs:"; outputWidth "Output width:"; outputBinaryPt "Output binary point position:"; outputArithmeticType "Output arithmetic type (ufix=0, fix=1, bool=2):"; show_format "Print format string?"; outputToWorkspace "Output to workspace?"; variablePrefix "Variable name prefix:"; outputToModelAsWell "Output to model as well?"
      mask help:
      | Expands a 'bus' made using a bus_create or Xilinx
      | concat block.
      | The input will be divided into the specified number
      | of outputs with the specified arithmetic types.
      | Divisions are made from most significant bit.
      mask init: same as pfb_core_snbxfft/pfb/pfb_fir_generic/bus_expand
      settings: AttributesFormatString=12 outputs: b,b,b,b,b,b,b,b,b,b,b,b,
      mask TypeOptions mode: divisions of equal size | divisions of arbitrary size
      mask Callback mode: bus_expand_callback();
      mask Callback outputWidth: bus_expand_callback();
      mask Callback outputToWorkspace: bus_expand_callback();
  dout : Outport
  wires:
  dout_compress/1(bus_out) -> dout/1
  del12/1 -> dout_compress/12(in12)
  del11/1 -> dout_compress/11(in11)
  del10/1 -> dout_compress/10(in10)
  del9/1 -> dout_compress/9(in9)
  del8/1 -> dout_compress/8(in8)
  del7/1 -> dout_compress/7(in7)
  del6/1 -> dout_compress/6(in6)
  del5/1 -> dout_compress/5(in5)
  del4/1 -> dout_compress/4(in4)
  del3/1 -> dout_compress/3(in3)
  del2/1 -> dout_compress/2(in2)
  del1/1 -> dout_compress/1(in1)
  en_expand/12(lsb_out1) -> del12/2
  din_expand/12(lsb_out1) -> del12/1
  en_expand/11(out2) -> del11/2
  din_expand/11(out2) -> del11/1
  en_expand/10(out3) -> del10/2
  din_expand/10(out3) -> del10/1
  en_expand/9(out4) -> del9/2
  din_expand/9(out4) -> del9/1
  en_expand/8(out5) -> del8/2
  din_expand/8(out5) -> del8/1
  en_expand/7(out6) -> del7/2
  din_expand/7(out6) -> del7/1
  en_expand/6(out7) -> del6/2
  din_expand/6(out7) -> del6/1
  en_expand/5(out8) -> del5/2
  din_expand/5(out8) -> del5/1
  en_expand/4(out9) -> del4/2
  din_expand/4(out9) -> del4/1
  en_expand/3(out10) -> del3/2
  din_expand/3(out10) -> del3/1
  en_expand/2(out11) -> del2/2
  din_expand/2(out11) -> del2/1
  en_expand/1(msb_out12) -> del1/2
  din_expand/1(msb_out12) -> del1/1
  en/1 -> en_expand/1(bus_in)
  din/1 -> din_expand/1(bus_in)

== system pfb_core_snbxfft/pfb/pfb_fir_generic/pfb_fir_taps/ddata1 ==
  din : Inport
  en : Inport  Port=2
  del{1..14} (14 alike) : xbsIndex_r4/Delay  rst=off  infoeditControl=Selection of Reset will increase slice count due to use of real FFs and instead of SRLs  en=on  latency=2  dbl_ovrd=off  reg_retiming=on  block_type=delay
  din_expand : Subsystem  AncestorBlock=casper_library_flow_control/bus_expand  mask(bus_expand){mode=divisions of arbitrary size, outputNum=1, outputWidth=[36  36  36  36  36  36  36  36  36  36  36  36  36  36], outputBinaryPt=[0  0  0  0  0  0  0  0  0  0  0  0  0  0], outputArithmeticType=[0  0  0  0  0  0  0  0  0  0  0  0  0  0], show_format=on, outputToWorkspace=off, variablePrefix=, outputToModelAsWell=on}
      mask prompts: outputNum "Number of outputs:"; outputWidth "Output width [msb ... lsb]:"; outputBinaryPt "Output binary point position [msb ... lsb]:"; outputArithmeticType "Output arithmetic type (ufix=0, fix=1, bool=2) [msb ... lsb]:"; show_format "Print format string?"; outputToWorkspace "Output to workspace?"; variablePrefix "Variable name prefix:"; outputToModelAsWell "Output to model as well?"
      mask help:
      | Expands a 'bus' made using a bus_create or Xilinx
      | concat block.
      | The input will be divided into the specified number
      | of outputs with the specified arithmetic types.
      | Divisions are made from most significant bit.
      mask init: same as pfb_core_snbxfft/pfb/pfb_fir_generic/bus_expand
      settings: AttributesFormatString=14 outputs: uf36.0,uf36.0,uf36.0,uf36.0,uf36.0,uf36.0,uf36.0,uf36.0,uf36.0,uf36.0,uf36.0,uf36.0,uf36.0,uf36.0,
      mask TypeOptions mode: divisions of equal size | divisions of arbitrary size
      mask Callback mode: bus_expand_callback();
      mask Callback outputWidth: bus_expand_callback();
      mask Callback outputToWorkspace: bus_expand_callback();
  dout_compress : Subsystem  AncestorBlock=casper_library_flow_control/bus_create  mask(bus_create){inputNum=14}
      mask prompts: inputNum "Number of inputs:"
      mask init:
      | bus_create_init(gcb,...
      |     'inputNum', inputNum);
  en_expand : Subsystem  AncestorBlock=casper_library_flow_control/bus_expand  mask(bus_expand){mode=divisions of equal size, outputNum=14, outputWidth=1, outputBinaryPt=0, outputArithmeticType=2, show_format=on, outputToWorkspace=off, variablePrefix=, outputToModelAsWell=on}
      mask prompts: outputNum "Number of outputs:"; outputWidth "Output width:"; outputBinaryPt "Output binary point position:"; outputArithmeticType "Output arithmetic type (ufix=0, fix=1, bool=2):"; show_format "Print format string?"; outputToWorkspace "Output to workspace?"; variablePrefix "Variable name prefix:"; outputToModelAsWell "Output to model as well?"
      mask help:
      | Expands a 'bus' made using a bus_create or Xilinx
      | concat block.
      | The input will be divided into the specified number
      | of outputs with the specified arithmetic types.
      | Divisions are made from most significant bit.
      mask init: same as pfb_core_snbxfft/pfb/pfb_fir_generic/bus_expand
      settings: AttributesFormatString=14 outputs: b,b,b,b,b,b,b,b,b,b,b,b,b,b,
      mask TypeOptions mode: divisions of equal size | divisions of arbitrary size
      mask Callback mode: bus_expand_callback();
      mask Callback outputWidth: bus_expand_callback();
      mask Callback outputToWorkspace: bus_expand_callback();
  dout : Outport
  wires:
  dout_compress/1(bus_out) -> dout/1
  del14/1 -> dout_compress/14(in14)
  del13/1 -> dout_compress/13(in13)
  del12/1 -> dout_compress/12(in12)
  del11/1 -> dout_compress/11(in11)
  del10/1 -> dout_compress/10(in10)
  del9/1 -> dout_compress/9(in9)
  del8/1 -> dout_compress/8(in8)
  del7/1 -> dout_compress/7(in7)
  del6/1 -> dout_compress/6(in6)
  del5/1 -> dout_compress/5(in5)
  del4/1 -> dout_compress/4(in4)
  del3/1 -> dout_compress/3(in3)
  del2/1 -> dout_compress/2(in2)
  del1/1 -> dout_compress/1(in1)
  en_expand/14(lsb_out1) -> del14/2
  din_expand/14(lsb_out1) -> del14/1
  en_expand/13(out2) -> del13/2
  din_expand/13(out2) -> del13/1
  en_expand/12(out3) -> del12/2
  din_expand/12(out3) -> del12/1
  en_expand/11(out4) -> del11/2
  din_expand/11(out4) -> del11/1
  en_expand/10(out5) -> del10/2
  din_expand/10(out5) -> del10/1
  en_expand/9(out6) -> del9/2
  din_expand/9(out6) -> del9/1
  en_expand/8(out7) -> del8/2
  din_expand/8(out7) -> del8/1
  en_expand/7(out8) -> del7/2
  din_expand/7(out8) -> del7/1
  en_expand/6(out9) -> del6/2
  din_expand/6(out9) -> del6/1
  en_expand/5(out10) -> del5/2
  din_expand/5(out10) -> del5/1
  en_expand/4(out11) -> del4/2
  din_expand/4(out11) -> del4/1
  en_expand/3(out12) -> del3/2
  din_expand/3(out12) -> del3/1
  en_expand/2(out13) -> del2/2
  din_expand/2(out13) -> del2/1
  en_expand/1(msb_out14) -> del1/2
  din_expand/1(msb_out14) -> del1/1
  en/1 -> en_expand/1(bus_in)
  din/1 -> din_expand/1(bus_in)
